simulink model "ukol1_2_porovnani"  (R2024b)
settings: Solver=VariableStepAuto  StartTime=0.0  StopTime=40000  RelTol=1e-3
settings Model: Creator=jirka  LastModifiedBy=jirka

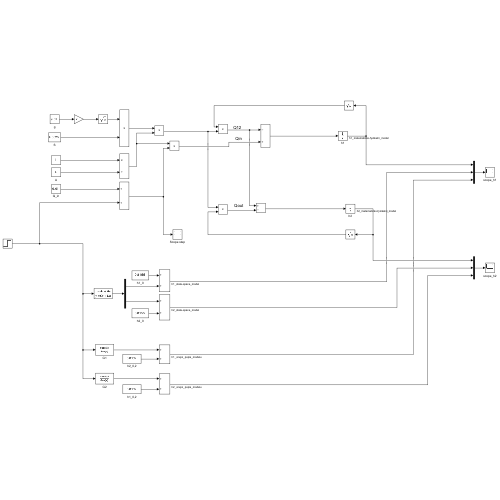
[thumbnail: Simulink's stored preview of the top-level diagram]
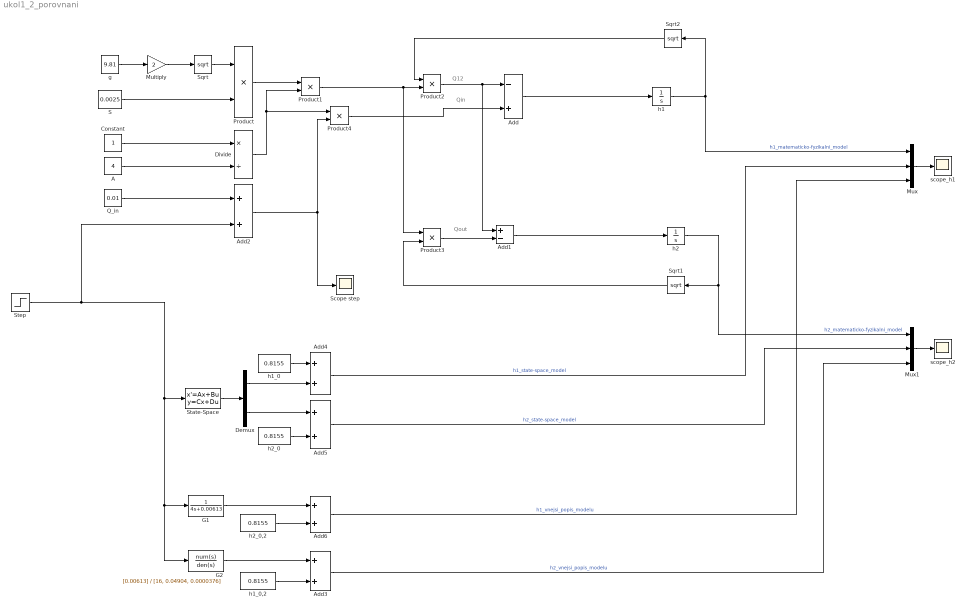
== system ukol1_2_porovnani ==
  note: Q12
  note: Qin
  note: Qout
  A : Constant  Value=4
  Add : Sum  Inputs=-+
  Add1 : Sum  Inputs=+-
  Add{2..6} (5 alike) : Sum
  Constant : Constant
  Demux : Demux  Outputs=2
  Divide : Product  Inputs=*/
  G1 : TransferFcn  Denominator=[4, 0.00613]
  G2 : TransferFcn  Numerator=[0.00613]  Denominator=[16, 0.04904, 0.0000376]
  Multiply : Gain  Gain=2
  Mux : Mux  Inputs=3
  Mux1 : Mux  Inputs=3
  Product{,1..4} (5 alike) : Product
  Q_in : Constant  Value=0.01
  S : Constant  Value=0.0025
  Scope step : Scope
  Sqrt : Sqrt
  Sqrt1 : Sqrt
  Sqrt2 : Sqrt
  State-Space : StateSpace  A=[-0.00153 0; 0.00153 -0.00153]  B=[0.25; 0]  C=[1 0; 0 1]  D=[0; 0]  InitialCondition=0
  Step : Step  Time=20000  After=0.005  SampleTime=0
  g : Constant  Value=9.81
  h1 : Integrator  InitialCondition=0.82
  h1_0 : Constant  Value=0.8155
  h1_0,2 : Constant  Value=0.8155
  h2 : Integrator  InitialCondition=0.82
  h2_0 : Constant  Value=0.8155
  h2_0,2 : Constant  Value=0.8155
  scope_h1 : Scope
  scope_h2 : Scope
  wires:
  Product4/1 -> Add/2
  Sqrt/1 -> Product/1
  Divide/1 -> Product4/1, Product1/2
  Product/1 -> Product1/1
  Multiply/1 -> Sqrt/1
  g/1 -> Multiply/1
  Product2/1 -> Add/1, Add1/1
  Q_in/1 -> Add2/1
  h2/1 -> Mux1/1, Sqrt1/1  "h2_matematicko-fyzikalni_model"
  Add2/1 -> Product4/2, Scope step/1
  Add/1 -> h1/1
  h1/1 -> Sqrt2/1, Mux/1  "h1_matematicko-fyzikalni_model"
  Constant/1 -> Divide/1
  Product1/1 -> Product3/1, Product2/2
  Product3/1 -> Add1/2
  Add1/1 -> h2/1
  Sqrt1/1 -> Product3/2
  A/1 -> Divide/2
  Sqrt2/1 -> Product2/1
  S/1 -> Product/2
  h2_0/1 -> Add5/2
  G2/1 -> Add3/1
  h1_0,2/1 -> Add3/2
  h1_0/1 -> Add4/1
  State-Space/1 -> Demux/1
  Step/1 -> G2/1, G1/1, State-Space/1, Add2/2
  Add4/1 -> Mux/2  "h1_state-space_model"
  Add5/1 -> Mux1/2  "h2_state-space_model"
  Demux/1 -> Add4/2
  Demux/2 -> Add5/1
  G1/1 -> Add6/1
  Add3/1 -> Mux1/3  "h2_vnejsi_popis_modelu"
  Add6/1 -> Mux/3  "h1_vnejsi_popis_modelu"
  h2_0,2/1 -> Add6/2
  Mux/1 -> scope_h1/1
  Mux1/1 -> scope_h2/1
